simulink model "fxpdemo_approx"  (Simulink 5.0)
settings: Solver=FixedStepDiscrete  StartTime=0.0  StopTime=1  FixedStep=0.01  RelTol=1e-3
InitFcn:
  | if ~exist('xuneven') | ~exist('yuneven') | ~exist('xeven') | ~exist('yeven') | ~exist('xpow2') | ~exist('ypow2'), fxpdemo_approx_sin, end
undefined symbols (not defined in the file or in its folder): xeven, xpow2, xuneven, yeven, ypow2, yuneven
libraries: fixpt_lib_4 x2
settings Model: CovMetricSettings=d  MinMaxOverflowLogging=MinMaxAndOverflow  Creator=andyb  LastModifiedBy=andyb  ExtModeAutoUpdateStatusClock=off  TunableVars=xuneven,yeven,ypow2,yuneven  TunableVarsStorageClass=ExportedGlobal,ExportedGlobal,ExportedGlobal,ExportedGlobal  TunableVarsTypeQualifier=,,,  SaveTime=off  SaveOutput=off  ParameterDowncastMsg=warning  ParameterOverflowMsg=warning  ParameterPrecisionLossMsg=none  RTWInlineParameters=on  BooleanDataType=off  RTWOptions="-aEnforceIntegerDowncast=1 -aExtMode=0 -aExtModeTesting=0 -aFoldNonRolledExpr=1 -aForceParamTrailComments=0 -aGenRTModel=1 -aGenerateComments=1 -aGenerateReport=0 -aIgnoreCustomStorageClasses=1 -aIncHierarchyInIds=0 -aInlineInvariantSignals=1 -aLocalBlockOutputs=1 -aLogVarNameModifier=\"rt_\" -aRTWVerbose=1 -aRollThreshold=5 -aShowEliminatedStatements=1"

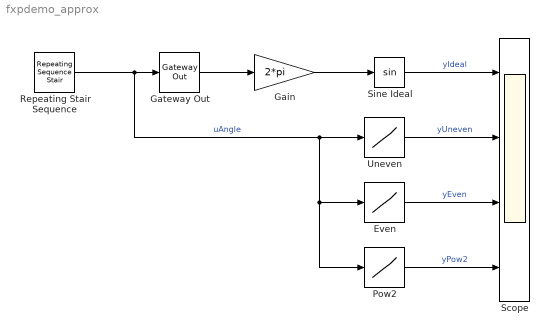
== system fxpdemo_approx ==
  Even : Lookup  InputValues=xeven  OutputValues=yeven  ShowAdditionalParam=on  LookUpMeth=Interpolation-Use End Values  OutDataTypeMode=Specify via dialog  OutScaling=2^-14
      settings: AttributesFormatString=Sine Approx
  Gain : Gain  Gain=2*pi  SaturateOnIntegerOverflow=on
  Gateway Out : fixpt_lib_4/Data Type/Gateway Out  OutRealWorld=Real World Value  OutBuiltInType=double  DoSatur=off
  Pow2 : Lookup  InputValues=xpow2  OutputValues=ypow2  ShowAdditionalParam=on  LookUpMeth=Interpolation-Use End Values  OutDataTypeMode=Specify via dialog  OutScaling=2^-14
      settings: AttributesFormatString=Sine Approx
  Repeating Stair Sequence : fixpt_lib_4/Sources/Repeating Sequence Stair  OutValues=linspace(0,0.25,100).'  tsamp=-1  OutputDataTypeScalingMode=Specify via dialog  OutDataType=ufix(16)  OutScaling=2^-14  ConRadixGroup=Use Specified Scaling
  Scope : Scope  NumInputPorts=4
      settings: TimeRange=1  YMin=0~0~0~0  YMax=1~1~1~1
  Sine Ideal : Trigonometry
  Uneven : Lookup  InputValues=xuneven  OutputValues=yuneven  ShowAdditionalParam=on  LookUpMeth=Interpolation-Use End Values  OutDataTypeMode=Specify via dialog  OutScaling=2^-14
      settings: AttributesFormatString=Sine Approx
  wires:
  Repeating Stair Sequence/1 -> Even/1, Pow2/1, Uneven/1, Gateway Out/1  "uAngle"
  Gain/1 -> Sine Ideal/1
  Gateway Out/1 -> Gain/1
  Sine Ideal/1 -> Scope/1  "yIdeal"
  Uneven/1 -> Scope/2  "yUneven"
  Even/1 -> Scope/3  "yEven"
  Pow2/1 -> Scope/4  "yPow2"
